simulink model "orbit3d"  (R2019b)
settings: Solver=ode4  StartTime=0.0  StopTime=7000  FixedStep=1  RelTol=1e-3
values from neighbouring files (symbols this model uses):
  initial_classical_comms = [comms_mean_sma ... (first row only)    [attitude3d_init.m]
  initial_classical_satellite = [satellite_sma ... (first row only)    [attitude3d_init.m]
  initial_classical_target = [target_mean_sma ... (first row only)    [attitude3d_init.m]
  P = 2 * pi / mean_motion    [attitude3d_init.m]
  target_mean_radius = mean_mars_radius    (= 3389500)    [attitude3d_init.m]
libraries: vrlib x2, simulink x1
settings Model: Creator=ggarrett  LastModifiedBy=ggarrett

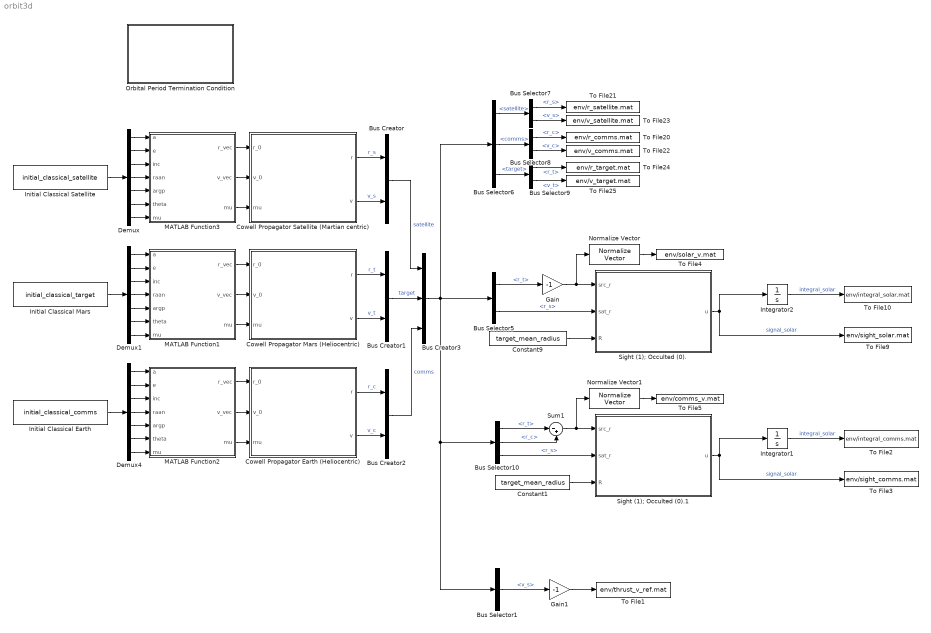
== system orbit3d ==
  Bus Creator : BusCreator  Inputs=2
  Bus Creator1 : BusCreator  Inputs=2
  Bus Creator2 : BusCreator  Inputs=2
  Bus Creator3 : BusCreator  Inputs=3
  Bus Selector1 : BusSelector  OutputSignals=satellite.v_s
  Bus Selector10 : BusSelector  OutputSignals=target.r_t,comms.r_c,satellite.r_s
  Bus Selector5 : BusSelector  OutputSignals=target.r_t,satellite.r_s
  Bus Selector6 : BusSelector  OutputSignals=satellite,comms,target
  Bus Selector7 : BusSelector  OutputSignals=r_s,v_s
  Bus Selector8 : BusSelector  OutputSignals=r_c,v_c
  Bus Selector9 : BusSelector  OutputSignals=r_t,v_t
  Constant1 : Constant  Value=target_mean_radius
  Constant9 : Constant  Value=target_mean_radius
  Cowell Propagator Earth (Heliocentric) : Subsystem
  Cowell Propagator Mars (Heliocentric) : Subsystem
  Cowell Propagator Satellite (Martian centric) : Subsystem
  Demux : Demux  Outputs=7
  Demux1 : Demux  Outputs=7
  Demux4 : Demux  Outputs=7
  Gain : Gain  Gain=-1
  Gain1 : Gain  Gain=-1
  Initial Classical Earth : Constant  Value=initial_classical_comms
  Initial Classical Mars : Constant  Value=initial_classical_target  VectorParams1D=off
  "Initial Classical Satellite " : Constant  Value=initial_classical_satellite
  Integrator1 : Integrator
  Integrator2 : Integrator
  MATLAB Function1 : MATLAB Function  TreatAsAtomicUnit=on
  MATLAB Function2 : MATLAB Function  TreatAsAtomicUnit=on
  MATLAB Function3 : MATLAB Function  TreatAsAtomicUnit=on
  Normalize Vector : vrlib/Utilities/Normalize Vector  maxzero=0
      settings: SourceProductName=Simulink
  Normalize Vector1 : vrlib/Utilities/Normalize Vector  maxzero=0
      settings: SourceProductName=Simulink
  Orbital Period Termination Condition : Subsystem
  Sight (1); Occulted (0). : MATLAB Function  TreatAsAtomicUnit=on
  Sight (1); Occulted (0).1 : MATLAB Function  TreatAsAtomicUnit=on
  Sum1 : Sum  Inputs=|-+
  To File1 : ToFile  Filename=env/thrust_v_ref.mat  SaveFormat=Timeseries
  To File10 : ToFile  Filename=env/integral_solar.mat  SaveFormat=Timeseries
  To File2 : ToFile  Filename=env/integral_comms.mat  SaveFormat=Timeseries
  To File20 : ToFile  Filename=env/r_comms.mat  SaveFormat=Timeseries
  To File21 : ToFile  Filename=env/r_satellite.mat  SaveFormat=Timeseries
  To File22 : ToFile  Filename=env/v_comms.mat  SaveFormat=Timeseries
  To File23 : ToFile  Filename=env/v_satellite.mat  SaveFormat=Timeseries
  To File24 : ToFile  Filename=env/r_target.mat  SaveFormat=Timeseries
  To File25 : ToFile  Filename=env/v_target.mat  SaveFormat=Timeseries
  To File3 : ToFile  Filename=env/sight_comms.mat  SaveFormat=Timeseries
  To File4 : ToFile  Filename=env/solar_v.mat  SaveFormat=Timeseries
  To File5 : ToFile  Filename=env/comms_v.mat  SaveFormat=Timeseries
  To File9 : ToFile  Filename=env/sight_solar.mat  SaveFormat=Timeseries
  wires:
  Initial Classical Mars/1 -> Demux1/1
  Demux/7 -> MATLAB Function3/7("mu ")
  Demux1/2 -> MATLAB Function1/2(e)
  Demux/5 -> MATLAB Function3/5(argp)
  Demux/4 -> MATLAB Function3/4(raan)
  "Initial Classical Satellite "/1 -> Demux/1
  Demux/1 -> MATLAB Function3/1(a)
  Demux/6 -> MATLAB Function3/6(theta)
  Demux1/1 -> MATLAB Function1/1(a)
  Demux1/4 -> MATLAB Function1/4(raan)
  Demux/3 -> MATLAB Function3/3(inc)
  Demux1/3 -> MATLAB Function1/3(inc)
  Demux1/5 -> MATLAB Function1/5(argp)
  Demux/2 -> MATLAB Function3/2(e)
  Demux1/6 -> MATLAB Function1/6(theta)
  Demux1/7 -> MATLAB Function1/7("mu ")
  Demux4/7 -> MATLAB Function2/7("mu ")
  Demux4/2 -> MATLAB Function2/2(e)
  Demux4/1 -> MATLAB Function2/1(a)
  Initial Classical Earth/1 -> Demux4/1
  Demux4/5 -> MATLAB Function2/5(argp)
  Demux4/3 -> MATLAB Function2/3(inc)
  Demux4/6 -> MATLAB Function2/6(theta)
  Demux4/4 -> MATLAB Function2/4(raan)
  MATLAB Function2/1(r_vec) -> Cowell Propagator Earth (Heliocentric)/1(r_0)
  MATLAB Function2/2(v_vec) -> Cowell Propagator Earth (Heliocentric)/2(v_0)
  MATLAB Function2/3(mu) -> Cowell Propagator Earth (Heliocentric)/3(mu)
  MATLAB Function1/1(r_vec) -> Cowell Propagator Mars (Heliocentric)/1(r_0)
  MATLAB Function1/2(v_vec) -> Cowell Propagator Mars (Heliocentric)/2(v_0)
  MATLAB Function1/3(mu) -> Cowell Propagator Mars (Heliocentric)/3(mu)
  MATLAB Function3/3(mu) -> Cowell Propagator Satellite (Martian centric)/3(mu)
  MATLAB Function3/2(v_vec) -> Cowell Propagator Satellite (Martian centric)/2(v_0)
  MATLAB Function3/1(r_vec) -> Cowell Propagator Satellite (Martian centric)/1(r_0)
  Constant9/1 -> Sight (1); Occulted (0)./3(R)
  Sight (1); Occulted (0)./1(u) -> To File9/1, Integrator2/1  "signal_solar"
  Integrator2/1 -> To File10/1  "integral_solar"
  Cowell Propagator Satellite (Martian centric)/1(r) -> Bus Creator/1  "r_s"
  Cowell Propagator Satellite (Martian centric)/2(v) -> Bus Creator/2  "v_s"
  Cowell Propagator Earth (Heliocentric)/1(r) -> Bus Creator2/1  "r_c"
  Cowell Propagator Earth (Heliocentric)/2(v) -> Bus Creator2/2  "v_c"
  Cowell Propagator Mars (Heliocentric)/2(v) -> Bus Creator1/2  "v_t"
  Cowell Propagator Mars (Heliocentric)/1(r) -> Bus Creator1/1  "r_t"
  Bus Creator/1 -> Bus Creator3/1  "satellite"
  Bus Creator1/1 -> Bus Creator3/2  "target"
  Bus Creator2/1 -> Bus Creator3/3  "comms"
  Bus Creator3/1 -> Bus Selector6/1, Bus Selector5/1, Bus Selector1/1, Bus Selector10/1
  Bus Selector7/1 -> To File21/1  "<r_s>"
  Bus Selector9/1 -> To File24/1  "<r_t>"
  Bus Selector8/1 -> To File20/1  "<r_c>"
  Bus Selector6/3 -> Bus Selector9/1  "<target>"
  Bus Selector7/2 -> To File23/1  "<v_s>"
  Bus Selector6/2 -> Bus Selector8/1  "<comms>"
  Bus Selector6/1 -> Bus Selector7/1  "<satellite>"
  Bus Selector8/2 -> To File22/1  "<v_c>"
  Bus Selector9/2 -> To File25/1  "<v_t>"
  Bus Selector5/2 -> Sight (1); Occulted (0)./2(sat_r)  "<r_s>"
  Bus Selector5/1 -> Gain/1  "<r_t>"
  Gain/1 -> Normalize Vector/1, Sight (1); Occulted (0)./1(src_r)
  Sight (1); Occulted (0).1/1(u) -> To File3/1, Integrator1/1  "signal_solar"
  Bus Selector10/1 -> Sum1/1  "<r_t>"
  Sum1/1 -> Normalize Vector1/1, Sight (1); Occulted (0).1/1(src_r)
  Bus Selector10/3 -> Sight (1); Occulted (0).1/2(sat_r)  "<r_s>"
  Integrator1/1 -> To File2/1  "integral_solar"
  Constant1/1 -> Sight (1); Occulted (0).1/3(R)
  Bus Selector10/2 -> Sum1/2  "<r_c>"
  Normalize Vector/1 -> To File4/1
  Normalize Vector1/1 -> To File5/1
  Gain1/1 -> To File1/1
  Bus Selector1/1 -> Gain1/1  "<v_s>"

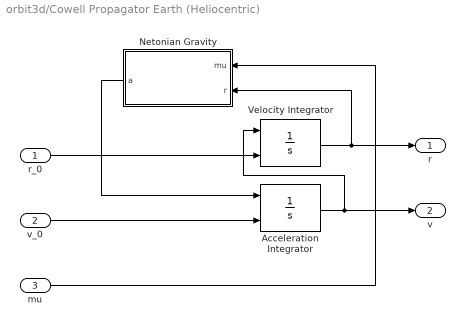
== system orbit3d/Cowell Propagator Earth (Heliocentric) ==
  r_0 : Inport
  v_0 : Inport  Port=2
  mu : Inport  Port=3
  Acceleration Integrator : Integrator  InitialConditionSource=external
  Netonian Gravity : MATLAB Function  TreatAsAtomicUnit=on
  Velocity Integrator : Integrator  InitialConditionSource=external
  r : Outport
  v : Outport  Port=2
  wires:
  Acceleration Integrator/1 -> v/1, Velocity Integrator/1
  v_0/1 -> Acceleration Integrator/2
  Velocity Integrator/1 -> r/1, Netonian Gravity/2(r)
  Netonian Gravity/1(a) -> Acceleration Integrator/1
  r_0/1 -> Velocity Integrator/2
  mu/1 -> Netonian Gravity/1(mu)

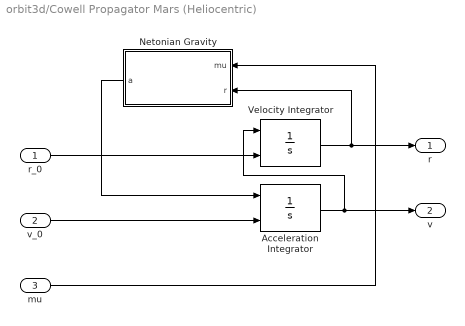
== system orbit3d/Cowell Propagator Mars (Heliocentric) ==
  r_0 : Inport
  v_0 : Inport  Port=2
  mu : Inport  Port=3
  Acceleration Integrator : Integrator  InitialConditionSource=external
  Netonian Gravity : MATLAB Function  TreatAsAtomicUnit=on
  Velocity Integrator : Integrator  InitialConditionSource=external
  r : Outport
  v : Outport  Port=2
  wires:
  Acceleration Integrator/1 -> v/1, Velocity Integrator/1
  v_0/1 -> Acceleration Integrator/2
  Velocity Integrator/1 -> r/1, Netonian Gravity/2(r)
  Netonian Gravity/1(a) -> Acceleration Integrator/1
  r_0/1 -> Velocity Integrator/2
  mu/1 -> Netonian Gravity/1(mu)

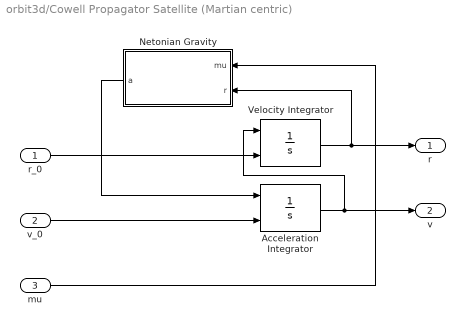
== system orbit3d/Cowell Propagator Satellite (Martian centric) ==
  r_0 : Inport
  v_0 : Inport  Port=2
  mu : Inport  Port=3
  Acceleration Integrator : Integrator  InitialConditionSource=external
  Netonian Gravity : MATLAB Function  TreatAsAtomicUnit=on
  Velocity Integrator : Integrator  InitialConditionSource=external
  r : Outport
  v : Outport  Port=2
  wires:
  Acceleration Integrator/1 -> v/1, Velocity Integrator/1
  v_0/1 -> Acceleration Integrator/2
  Velocity Integrator/1 -> r/1, Netonian Gravity/2(r)
  Netonian Gravity/1(a) -> Acceleration Integrator/1
  r_0/1 -> Velocity Integrator/2
  mu/1 -> Netonian Gravity/1(mu)

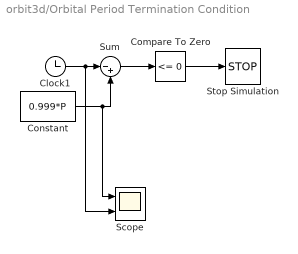
== system orbit3d/Orbital Period Termination Condition ==
  Clock1 : Clock
  Compare To Zero : simulink/Logic and Bit Operations/Compare To Zero  relop=<=  OutDataTypeStr=boolean
  Constant : Constant  Value=0.999*P
  Scope : Scope  NumInputPorts=2
  Stop Simulation : Stop
  Sum : Sum  Inputs=|-+
  wires:
  Constant/1 -> Scope/1, Sum/2
  Clock1/1 -> Scope/2, Sum/1
  Sum/1 -> Compare To Zero/1
  Compare To Zero/1 -> Stop Simulation/1

== matlab function orbit3d/MATLAB Function3 ==
  data: a input; r_vec output; e input; inc input; raan input; argp input; theta input; mu input; v_vec output; mu output
function [r_vec,v_vec, mu] = coe2rv(a, e, inc, raan, argp, theta, mu)
    cos_raan = cos(raan);
    sin_raan = sin(raan);
    cos_argp = cos(argp);
    sin_argp = sin(argp);
    cos_inc = cos(inc);
    sin_inc = sin(inc);
    r = a * (1 - e ^ 2) / (1.0 + e * cos(theta));

    l1 = (+cos_raan * cos_argp - sin_raan * sin_argp * cos_inc);
    l2 = (-cos_raan * sin_argp - sin_raan * cos_argp * cos_inc);
    m1 = (+sin_raan * cos_argp + cos_raan * sin_argp * cos_inc);
    m2 = (-sin_raan * sin_argp + cos_raan * cos_argp * cos_inc);
    n1 = sin_argp * sin_inc;
    n2 = cos_argp * sin_inc;

    aux = [r * cos(theta); r * sin(theta)];
    transformation = [l1, l2;...
                      m1, m2;...
                      n1, n2];

    % Position
    xyz = transformation * aux;
    x = xyz(1);
    y = xyz(2);
    z = xyz(3);

    % Velocity
    H = sqrt(mu * a * (1 - e ^ 2));
    v_x = mu / H * (-l1 * sin(theta) + l2 * (e + cos(theta)));
    v_y = mu / H * (-m1 * sin(theta) + m2 * (e + cos(theta)));
    v_z = mu / H * (-n1 * sin(theta) + n2 * (e + cos(theta)));
    r_vec = [x; y; z];
    v_vec = [v_x; v_y; v_z];
end

== matlab function orbit3d/Cowell Propagator Earth (Heliocentric)/Netonian Gravity ==
  data: mu input; r input; a output
function a = newtonGrav(mu, r)

a = -(mu / norm(r)^3) * r;

== matlab function orbit3d/MATLAB Function2 ==
  data: a input; r_vec output; e input; inc input; raan input; argp input; theta input; mu input; v_vec output; mu output
function [r_vec,v_vec, mu] = coe2rv(a, e, inc, raan, argp, theta, mu)
    cos_raan = cos(raan);
    sin_raan = sin(raan);
    cos_argp = cos(argp);
    sin_argp = sin(argp);
    cos_inc = cos(inc);
    sin_inc = sin(inc);
    r = a * (1 - e ^ 2) / (1.0 + e * cos(theta));

    l1 = (+cos_raan * cos_argp - sin_raan * sin_argp * cos_inc);
    l2 = (-cos_raan * sin_argp - sin_raan * cos_argp * cos_inc);
    m1 = (+sin_raan * cos_argp + cos_raan * sin_argp * cos_inc);
    m2 = (-sin_raan * sin_argp + cos_raan * cos_argp * cos_inc);
    n1 = sin_argp * sin_inc;
    n2 = cos_argp * sin_inc;

    aux = [r * cos(theta); r * sin(theta)];
    transformation = [l1, l2;...
                      m1, m2;...
                      n1, n2];

    % Position
    xyz = transformation * aux;
    x = xyz(1);
    y = xyz(2);
    z = xyz(3);

    % Velocity
    H = sqrt(mu * a * (1 - e ^ 2));
    v_x = mu / H * (-l1 * sin(theta) + l2 * (e + cos(theta)));
    v_y = mu / H * (-m1 * sin(theta) + m2 * (e + cos(theta)));
    v_z = mu / H * (-n1 * sin(theta) + n2 * (e + cos(theta)));
    r_vec = [x; y; z];
    v_vec = [v_x; v_y; v_z];
end

== matlab function orbit3d/MATLAB Function1 ==
  data: a input; r_vec output; e input; inc input; raan input; argp input; theta input; mu input; v_vec output; mu output
function [r_vec,v_vec, mu] = coe2rv(a, e, inc, raan, argp, theta, mu)
    cos_raan = cos(raan);
    sin_raan = sin(raan);
    cos_argp = cos(argp);
    sin_argp = sin(argp);
    cos_inc = cos(inc);
    sin_inc = sin(inc);
    r = a * (1 - e ^ 2) / (1.0 + e * cos(theta));

    l1 = (+cos_raan * cos_argp - sin_raan * sin_argp * cos_inc);
    l2 = (-cos_raan * sin_argp - sin_raan * cos_argp * cos_inc);
    m1 = (+sin_raan * cos_argp + cos_raan * sin_argp * cos_inc);
    m2 = (-sin_raan * sin_argp + cos_raan * cos_argp * cos_inc);
    n1 = sin_argp * sin_inc;
    n2 = cos_argp * sin_inc;

    aux = [r * cos(theta); r * sin(theta)];
    transformation = [l1, l2;...
                      m1, m2;...
                      n1, n2];

    % Position
    xyz = transformation * aux;
    x = xyz(1);
    y = xyz(2);
    z = xyz(3);

    % Velocity
    H = sqrt(mu * a * (1 - e ^ 2));
    v_x = mu / H * (-l1 * sin(theta) + l2 * (e + cos(theta)));
    v_y = mu / H * (-m1 * sin(theta) + m2 * (e + cos(theta)));
    v_z = mu / H * (-n1 * sin(theta) + n2 * (e + cos(theta)));
    r_vec = [x; y; z];
    v_vec = [v_x; v_y; v_z];
end

== matlab function orbit3d/Cowell Propagator Mars (Heliocentric)/Netonian Gravity ==
  data: mu input; r input; a output
function a = newtonGrav(mu, r)

a = -(mu / norm(r)^3) * r;

== matlab function orbit3d/Cowell Propagator Satellite (Martian centric)/Netonian Gravity ==
  data: mu input; r input; a output
function a = newtonGrav(mu, r)

a = -(mu / norm(r)^3) * r;

== matlab function orbit3d/Sight (1); Occulted (0). ==
  data: src_r input; u output; sat_r input; R input
function u = sight_function(src_r, sat_r, R)
% Parameters
% ----------
% src_v : double, shape=(1,3)
%   source vector which is being checked for occultation by
%   planet of radius rad_p. Origin of vector is center of planet.
% sat_r : double, shape=(1,3)
%   inertial vector of satellite orbiting planet.
% R : double
%   radius of the planet being orbited.
spacecraft_h = norm(sat_r) - R; % Calculate spacecraft h.
src_v = src_r/norm(src_r);      % Source unit vector.
sat_v = sat_r/norm(sat_r);      % Satellite unit vector.
cos_phi = dot(src_v, sat_v);
a_sin_phi = (R + spacecraft_h) * sin(acos(cos_phi));
if (cos_phi < 0) && (a_sin_phi <R)
    u=0;   % Occulted (signal is blocked).
else
    u=1;   % Not occulted (allows signal to pass).
end

== matlab function orbit3d/Sight (1); Occulted (0).1 ==
  data: src_r input; u output; sat_r input; R input
function u = sight_function(src_r, sat_r, R)
% Parameters
% ----------
% src_v : double, shape=(1,3)
%   source vector which is being checked for occultation by
%   planet of radius rad_p. Origin of vector is center of planet.
% sat_r : double, shape=(1,3)
%   inertial vector of satellite orbiting planet.
% R : double
%   radius of the planet being orbited.
spacecraft_h = norm(sat_r) - R; % Calculate spacecraft h.
src_v = src_r/norm(src_r);      % Source unit vector.
sat_v = sat_r/norm(sat_r);      % Satellite unit vector.
cos_phi = dot(src_v, sat_v);
a_sin_phi = (R + spacecraft_h) * sin(acos(cos_phi));
if (cos_phi < 0) && (a_sin_phi <R)
    u=0;   % Occulted (signal is blocked).
else
    u=1;   % Not occulted (allows signal to pass).
end
